simulink library "thrNodeMass_ul"  (R2018b)
settings: Solver=VariableStepAuto  StartTime=0.0  StopTime=10.0  RelTol=1e-3
settings Model: Creator=asiddiq2  LastModifiedBy=mcobb

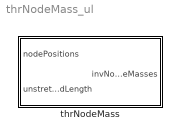
== system thrNodeMass_ul ==
  thrNodeMass : Subsystem  mask{tetherDensity=0, diameter=0}
      mask prompts: tetherDensity "Tether density"; diameter "Tether diameter"
      settings: MinAlgLoopOccurrences=on

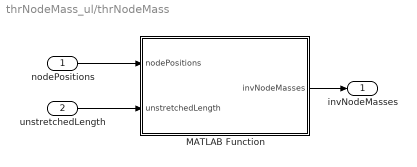
== system thrNodeMass_ul/thrNodeMass ==
  nodePositions : Inport
  unstretchedLength : Inport  Port=2
  MATLAB Function : MATLAB Function  TreatAsAtomicUnit=on
  invNodeMasses : Outport
  wires:
  MATLAB Function/1(invNodeMasses) -> invNodeMasses/1
  unstretchedLength/1 -> MATLAB Function/2(unstretchedLength)
  nodePositions/1 -> MATLAB Function/1(nodePositions)

== matlab function thrNodeMass_ul/thrNodeMass/MATLAB Function ==
  data: nodePositions input; invNodeMasses output; unstretchedLength input; tetherDensity parameter; diameter parameter
function invNodeMasses  = fcn(...
    nodePositions,unstretchedLength,...
    tetherDensity, diameter)

% In this notation, N is the number of nodes

% Length of each link 1xN-1
linkLengths = sqrt(sum(diff(nodePositions,1,2).^2));

% Total length of all links, assuming they're straight lines, scalar
numericalTotalLength = sum(linkLengths);

% Total volume based on unspooled length, scalar
analyticalTotalVol  = unstretchedLength*(pi/4)*diameter^2;

% Total mass, based on unspooled length, scalar
analyticalTotalMass = tetherDensity*analyticalTotalVol;

% Mass of each link, 1xN-1
linkMasses  = analyticalTotalMass*(linkLengths./numericalTotalLength);

% 1/mass for each node, 3xN (repmat so that we can multiply with force
% vectors concatenated into matrix later
invNodeMasses    = repmat(1./([linkMasses(1) linkMasses(1:end-1)+linkMasses(2:end) linkMasses(end)]/2),[3 1]);

end
